simulink model "simulink6"  (Simulink 5.0)
settings: Solver=FixedStepDiscrete  StartTime=0.0  StopTime=100.0  FixedStep=1  RelTol=1e-3
undefined symbols (not defined in the file): j, magnitude
settings Model: Creator=asteele  LastModifiedBy=stevel  ExtModeAutoUpdateStatusClock=off  BooleanDataType=off

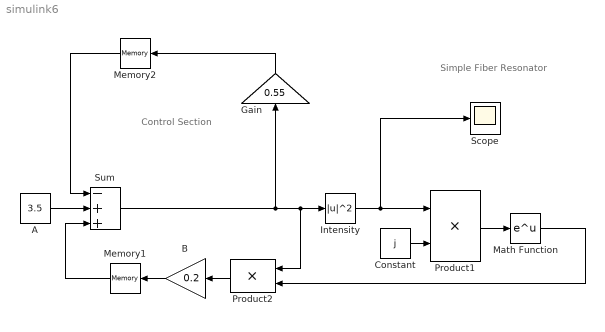
== system simulink6 ==
  note: Control Section
  note: Simple Fiber Resonator
  A : Constant  Value=3.5
  B : Gain  Orientation=left  Gain=0.2  SaturateOnIntegerOverflow=on
  Constant : Constant  Value=j
  Gain : Gain  Orientation=up  Gain=0.55  SaturateOnIntegerOverflow=on
  Intensity : Math  Operator=magnitude^2
  Math Function : Math
  Memory1 : Memory  Orientation=left
  Memory2 : Memory  Orientation=left
  Product1 : Product  SaturateOnIntegerOverflow=on  InputSameDT=on
  Product2 : Product  Orientation=left  SaturateOnIntegerOverflow=on  InputSameDT=on
  Scope : Scope
      settings: TimeRange=400000
  Sum : Sum  Inputs=-++  SaturateOnIntegerOverflow=on  InputSameDT=on
  wires:
  Intensity/1 -> Scope/1, Product1/1
  Product2/1 -> B/1
  B/1 -> Memory1/1
  Product1/1 -> Math Function/1
  Math Function/1 -> Product2/2
  Constant/1 -> Product1/2
  Gain/1 -> Memory2/1
  Memory1/1 -> Sum/3
  A/1 -> Sum/2
  Memory2/1 -> Sum/1
  Sum/1 -> Gain/1, Intensity/1, Product2/1
